simulink model "highpass"  (Simulink 7.7)
settings: Solver=ode45  StartTime=0.0  StopTime=(m-n)*sample  RelTol=1e-3
InitFcn:
  | %% DSPBuilder Start
  | alt_dspbuilder_update_model(bdroot)
  | %% DSPBuilder End
values from neighbouring files (symbols this model uses):
  sample = 10e-9    (= 1e-08)    [readdata.m]
undefined symbols (not defined in the file or in its folder): G, SOS
libraries: allblocks_alteradspbuilder2 x32, simulink x4
settings Model: Creator=Lyq  LastModifiedBy=xj

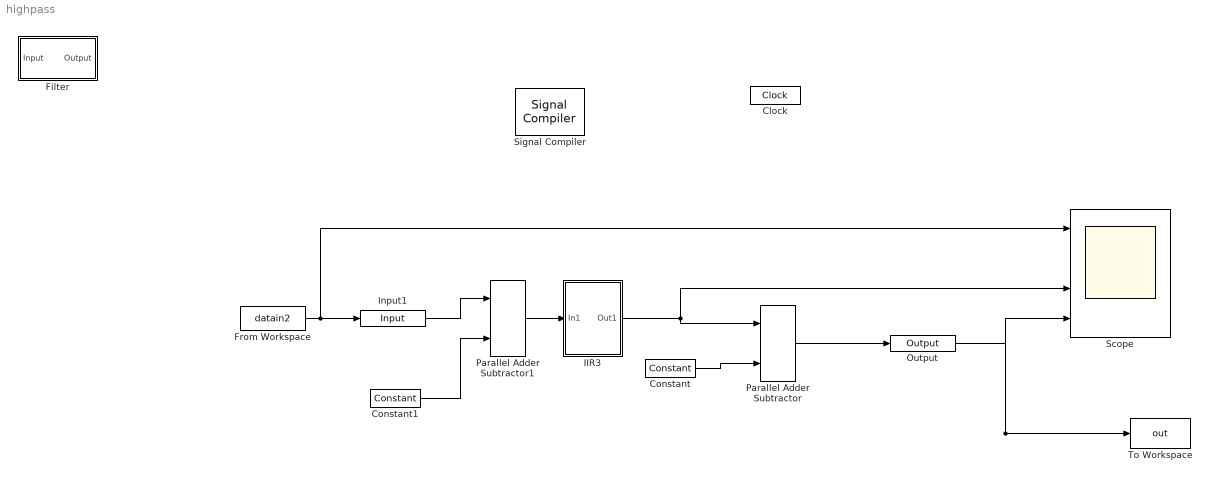
== system highpass ==
  Clock : allblocks_alteradspbuilder2/Clock  ClockPeriod=10  ClockPeriodUnit=ns  SampleTime=10e-9  ResetLatency=0  ResetRegisterCascadeDepth=0  SimulationStartCycle=5  PhaseOffset=0  Reset=aclr  ResetType=Active Low  Export=off
  Constant : allblocks_alteradspbuilder2/Constant  mask_cst=512  BusType=Unsigned Integer  bwl=10  bwr=0  roundMode=Truncate  satMode=Wrap  SpecifyClock=off  allowFloatingPointOverride=on  logOutputs=off  logFile=D:\highpass_Constant.fixedpointlog
  Constant1 : allblocks_alteradspbuilder2/Constant  mask_cst=512  BusType=Unsigned Integer  bwl=10  bwr=0  roundMode=Truncate  satMode=Wrap  SpecifyClock=off  allowFloatingPointOverride=on  logOutputs=off  logFile=D:\highpass_Constant1.fixedpointlog
  Filter : Subsystem  Tag=FilterWizardSubSystem
      settings: ErrorFcn=dspFilterRealizedInBasicElemsAlgLoopErrFcnCallback
  From Workspace : FromWorkspace  VariableName=datain2  SampleTime=sample
  IIR3 : Subsystem
  Input1 : allblocks_alteradspbuilder2/Input  iofile=F:\matlab\DSPbuilder\HighPass(1Mfc-100fs)\tb_highpass\highpass_Input1.salt  BusType=Unsigned Integer  bwl=10  bwr=5  SpecifyClock=off  PORTTYPE=Input  externalType=Inferred  allowFloatingPointOverride=on  logOutputs=off
  Output : allblocks_alteradspbuilder2/Output  iofile=F:\matlab\DSPbuilder\HighPass(1Mfc-100fs)\tb_highpass\highpass_Output.capture  BusType=Unsigned Integer  bwl=10  bwr=0  externalType=Inferred  PORTTYPE=Output  allowFloatingPointOverride=on  logOutputs=off
  Parallel Adder Subtractor : allblocks_alteradspbuilder2/Parallel Adder Subtractor  number_of_inputs=2  direction=+  use_pipeline=on  pipeline_display=1  phase_selection=1  use_ena=off  use_aclr=off  allowFloatingPointOverride=on  logOutputs=off  logFile=F:\matlab\DSPbuilder\bandpass(1-10M)\tb_bandpass\highpass_Parallel+Adder+Subtractor.fixedpointlog
  Parallel Adder Subtractor1 : allblocks_alteradspbuilder2/Parallel Adder Subtractor  number_of_inputs=2  direction=+-  use_pipeline=on  pipeline_display=1  phase_selection=1  use_ena=off  use_aclr=off  allowFloatingPointOverride=on  logOutputs=off  logFile=F:\matlab\DSPbuilder\bandpass(1-10M)\tb_bandpass\highpass_Parallel+Adder+Subtractor1.fixedpointlog
  Scope : Scope  NumInputPorts=4
      settings: TimeRange=3.839999999999997e-006  YMin=-30000~-30000~-40000~-40000  YMax=30000~30000~40000~40000  MaxDataPoints=50000  SampleInput=on
  Signal Compiler : allblocks_alteradspbuilder2/Signal Compiler  DeviceFamily=Cyclone III  DeviceName=AUTO  EnableSignalTap=off  SignalTapDepth=128  UseBoardBlock=off  StpUseDefaultClock=on  StpClock=Clock  ExportDir=F:\matlab\DSPbuilder\bandpass(1-10M)\HDL
  To Workspace : ToWorkspace  VariableName=out  SampleTime=-1  SaveFormat=Structure
  wires:
  From Workspace/1 -> Scope/1, Input1/1
  IIR3/1(Out1) -> Scope/3, Parallel Adder Subtractor/1
  Output/1 -> Scope/4, To Workspace/1
  Constant/1 -> Parallel Adder Subtractor/2
  Parallel Adder Subtractor/1 -> Output/1
  Parallel Adder Subtractor1/1 -> IIR3/1(In1)
  Input1/1 -> Parallel Adder Subtractor1/1
  Constant1/1 -> Parallel Adder Subtractor1/2

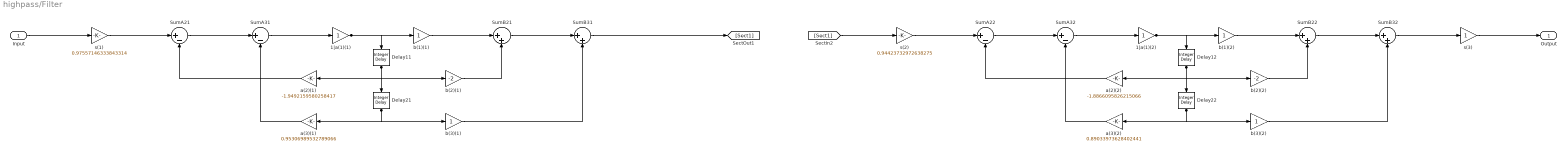
== system highpass/Filter ==
  Input : Inport
  1|a(1)(1) : Gain  ParamDataTypeStr=float('double')  RndMeth=Nearest  SaturateOnIntegerOverflow=on  OutDataTypeStr=Inherit: Same as input
  1|a(1)(2) : Gain  ParamDataTypeStr=float('double')  RndMeth=Nearest  SaturateOnIntegerOverflow=on  OutDataTypeStr=Inherit: Same as input
  Delay{11..12,21..22} (4 alike) : simulink/Discrete/Integer Delay  NumDelays=1  InputProcessing=Inherited  vinit=0  samptime=-1
  SumA{21..22,31..32} (4 alike) : Sum  Inputs=|+-  RndMeth=Nearest  SaturateOnIntegerOverflow=on  OutDataTypeStr=Inherit: Same as first input
  SumB{21..22,31..32} (4 alike) : Sum  Inputs=|++  RndMeth=Nearest  SaturateOnIntegerOverflow=on  OutDataTypeStr=Inherit: Same as first input
  a(2)(1) : Gain  Gain=-1.9492159580258417  ParamDataTypeStr=float('double')  RndMeth=Nearest  SaturateOnIntegerOverflow=on  OutDataTypeStr=Inherit: Same as input
  a(2)(2) : Gain  Gain=-1.8866095826215066  ParamDataTypeStr=float('double')  RndMeth=Nearest  SaturateOnIntegerOverflow=on  OutDataTypeStr=Inherit: Same as input
  a(3)(1) : Gain  Gain=0.95306989532789066  ParamDataTypeStr=float('double')  RndMeth=Nearest  SaturateOnIntegerOverflow=on  OutDataTypeStr=Inherit: Same as input
  a(3)(2) : Gain  Gain=0.89033973628402441  ParamDataTypeStr=float('double')  RndMeth=Nearest  SaturateOnIntegerOverflow=on  OutDataTypeStr=Inherit: Same as input
  b(1)(1) : Gain  ParamDataTypeStr=float('double')  RndMeth=Nearest  SaturateOnIntegerOverflow=on  OutDataTypeStr=Inherit: Same as input
  b(1)(2) : Gain  ParamDataTypeStr=float('double')  RndMeth=Nearest  SaturateOnIntegerOverflow=on  OutDataTypeStr=Inherit: Same as input
  b(2)(1) : Gain  Gain=-2  ParamDataTypeStr=float('double')  RndMeth=Nearest  SaturateOnIntegerOverflow=on  OutDataTypeStr=Inherit: Same as input
  b(2)(2) : Gain  Gain=-2  ParamDataTypeStr=float('double')  RndMeth=Nearest  SaturateOnIntegerOverflow=on  OutDataTypeStr=Inherit: Same as input
  b(3)(1) : Gain  ParamDataTypeStr=float('double')  RndMeth=Nearest  SaturateOnIntegerOverflow=on  OutDataTypeStr=Inherit: Same as input
  b(3)(2) : Gain  ParamDataTypeStr=float('double')  RndMeth=Nearest  SaturateOnIntegerOverflow=on  OutDataTypeStr=Inherit: Same as input
  s(1) : Gain  Gain=0.97557146333843314  ParamDataTypeStr=float('double')  RndMeth=Nearest  SaturateOnIntegerOverflow=on  OutDataTypeStr=Inherit: Same as input
  s(2) : Gain  Gain=0.94423732972638275  ParamDataTypeStr=float('double')  RndMeth=Nearest  SaturateOnIntegerOverflow=on  OutDataTypeStr=Inherit: Same as input
  s(3) : Gain  ParamDataTypeStr=float('double')  RndMeth=Nearest  SaturateOnIntegerOverflow=on  OutDataTypeStr=Inherit: Same as input
  Output : Outport
  wires:
  Input/1 -> s(1)/1
  s(1)/1 -> SumA21/1
  SumA21/1 -> SumA31/1
  SumA31/1 -> 1|a(1)(1)/1
  1|a(1)(1)/1 -> b(1)(1)/1, Delay11/1
  b(1)(1)/1 -> SumB21/1
  SumB21/1 -> SumB31/1
  SumB31/1 -> [Sect1]
  a(2)(1)/1 -> SumA21/2
  Delay11/1 -> a(2)(1)/1, b(2)(1)/1, Delay21/1
  b(2)(1)/1 -> SumB21/2
  a(3)(1)/1 -> SumA31/2
  Delay21/1 -> a(3)(1)/1, b(3)(1)/1
  b(3)(1)/1 -> SumB31/2
  [Sect1] -> s(2)/1
  s(2)/1 -> SumA22/1
  SumA22/1 -> SumA32/1
  SumA32/1 -> 1|a(1)(2)/1
  1|a(1)(2)/1 -> b(1)(2)/1, Delay12/1
  b(1)(2)/1 -> SumB22/1
  SumB22/1 -> SumB32/1
  SumB32/1 -> s(3)/1
  a(2)(2)/1 -> SumA22/2
  Delay12/1 -> a(2)(2)/1, b(2)(2)/1, Delay22/1
  b(2)(2)/1 -> SumB22/2
  a(3)(2)/1 -> SumA32/2
  Delay22/1 -> a(3)(2)/1, b(3)(2)/1
  b(3)(2)/1 -> SumB32/2
  s(3)/1 -> Output/1

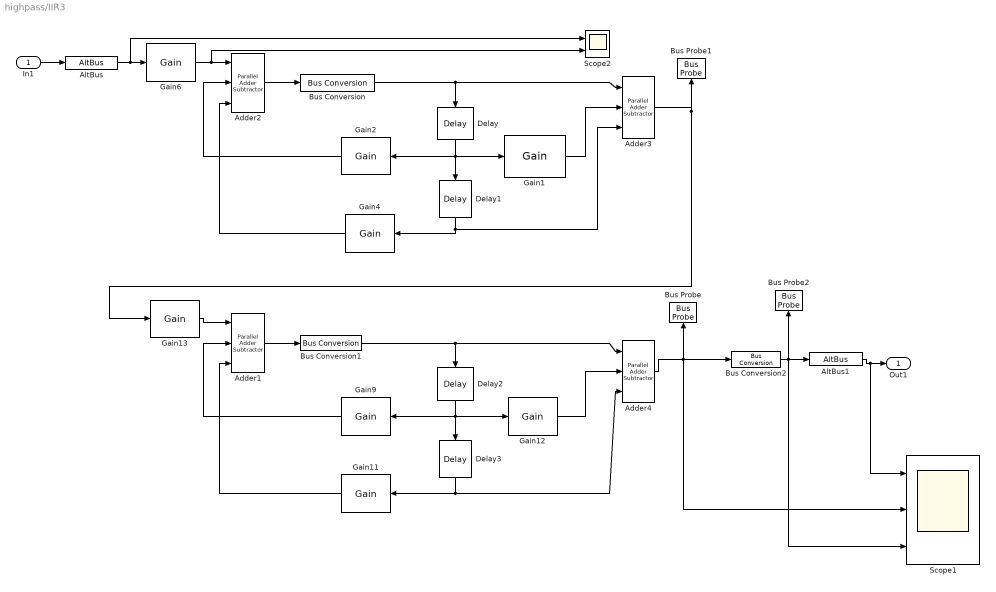
== system highpass/IIR3 ==
  In1 : Inport
  Adder1 : allblocks_alteradspbuilder2/Parallel Adder Subtractor  number_of_inputs=3  direction=+--  use_pipeline=off  pipeline_display=0  phase_selection=1  use_ena=off  use_aclr=off  allowFloatingPointOverride=on  logOutputs=off  logFile=D:\highpass_IIR3_Adder1.fixedpointlog
  Adder2 : allblocks_alteradspbuilder2/Parallel Adder Subtractor  number_of_inputs=3  direction=+--  use_pipeline=off  pipeline_display=0  phase_selection=1  use_ena=off  use_aclr=off  allowFloatingPointOverride=on  logOutputs=off  logFile=D:\highpass_IIR3_Adder2.fixedpointlog
  Adder3 : allblocks_alteradspbuilder2/Parallel Adder Subtractor  number_of_inputs=3  direction=+  use_pipeline=on  pipeline_display=2  phase_selection=1  use_ena=off  use_aclr=off  allowFloatingPointOverride=on  logOutputs=off  logFile=D:\highpass_IIR3_Adder3.fixedpointlog
  Adder4 : allblocks_alteradspbuilder2/Parallel Adder Subtractor  number_of_inputs=3  direction=+  use_pipeline=on  pipeline_display=2  phase_selection=1  use_ena=off  use_aclr=off  allowFloatingPointOverride=on  logOutputs=off  logFile=D:\highpass_IIR3_Adder4.fixedpointlog
  AltBus : allblocks_alteradspbuilder2/AltBus  BusType=Signed Integer  bwl=10  bwr=5  saturate=off  floatingPointInput=on  floatingPointOutput=on  logOutputs=off  logFile=D:\highpass_IIR3_AltBus.fixedpointlog
  AltBus1 : allblocks_alteradspbuilder2/AltBus  BusType=Signed Integer  bwl=10  bwr=5  saturate=on  floatingPointInput=on  floatingPointOutput=on  logOutputs=off  logFile=D:\highpass_IIR3_AltBus1.fixedpointlog
  Bus Conversion : allblocks_alteradspbuilder2/Bus Conversion  BusType=Signed Fractional  ibwl=20  ibwr=5  bwl=20  bwr=5  bitToConnectToOutputLSB=0  round=off  saturate=on  pipeline_display=0
  Bus Conversion1 : allblocks_alteradspbuilder2/Bus Conversion  BusType=Signed Fractional  ibwl=24  ibwr=5  bwl=24  bwr=5  bitToConnectToOutputLSB=0  round=off  saturate=on  pipeline_display=0
  Bus Conversion2 : allblocks_alteradspbuilder2/Bus Conversion  BusType=Signed Integer  ibwl=11  ibwr=1  bwl=10  bwr=1  bitToConnectToOutputLSB=0  round=off  saturate=on  pipeline_display=0
  Bus Probe : allblocks_alteradspbuilder2/Bus Probe  display=Maximum number of integer bits required during simulation  max_value=598.21875  min_value=-618.875  max_bits=11
  Bus Probe1 : allblocks_alteradspbuilder2/Bus Probe  display=Maximum number of integer bits required during simulation  max_value=755.5625  min_value=-665.78125  max_bits=11
  Bus Probe2 : allblocks_alteradspbuilder2/Bus Probe  display=Maximum number of integer bits required during simulation  max_value=511  min_value=-512  max_bits=10
  Delay : allblocks_alteradspbuilder2/Delay  pipeline=1  pipeline_display=1  ClockPhase=1  use_ena=off  use_sclr=off  allowFloatingPointOverride=on  logOutputs=off  logFile=D:\highpass_IIR3_Delay.fixedpointlog  use_init=off  reset_value=1
  Delay1 : allblocks_alteradspbuilder2/Delay  pipeline=1  pipeline_display=1  ClockPhase=1  use_ena=off  use_sclr=off  allowFloatingPointOverride=on  logOutputs=off  logFile=D:\highpass_IIR3_Delay1.fixedpointlog  use_init=off  reset_value=1
  Delay2 : allblocks_alteradspbuilder2/Delay  pipeline=1  pipeline_display=1  ClockPhase=1  use_ena=off  use_sclr=off  allowFloatingPointOverride=on  logOutputs=off  logFile=D:\highpass_IIR3_Delay2.fixedpointlog  use_init=off  reset_value=1
  Delay3 : allblocks_alteradspbuilder2/Delay  pipeline=1  pipeline_display=1  ClockPhase=1  use_ena=off  use_sclr=off  allowFloatingPointOverride=on  logOutputs=off  logFile=D:\highpass_IIR3_Delay3.fixedpointlog  use_init=off  reset_value=1
  Gain1 : allblocks_alteradspbuilder2/Gain  vgain=SOS(1,2)  BusType=Signed Fractional  bwl=2  bwr=16  pipeline=0  pipeline_display=0  allowFloatingPointOverride=on  logOutputs=off  logFile=D:\highpass_IIR3_Gain1.fixedpointlog  use_ena=off  use_aclr=off  lpm=off  MaskValue=1
  Gain11 : allblocks_alteradspbuilder2/Gain  vgain=SOS(2,6)  BusType=Signed Fractional  bwl=2  bwr=10  pipeline=0  pipeline_display=0  allowFloatingPointOverride=on  logOutputs=off  logFile=D:\highpass_IIR3_Gain11.fixedpointlog  use_ena=off  use_aclr=off  lpm=off  MaskValue=1
  Gain12 : allblocks_alteradspbuilder2/Gain  vgain=SOS(2,2)  BusType=Signed Integer  bwl=2  bwr=10  pipeline=0  pipeline_display=0  allowFloatingPointOverride=on  logOutputs=off  logFile=D:\highpass_IIR3_Gain12.fixedpointlog  use_ena=off  use_aclr=off  lpm=off  MaskValue=1
  Gain13 : allblocks_alteradspbuilder2/Gain  vgain=G(2)  BusType=Signed Fractional  bwl=2  bwr=10  pipeline=0  pipeline_display=0  allowFloatingPointOverride=on  logOutputs=off  logFile=D:\highpass_IIR3_Gain13.fixedpointlog  use_ena=off  use_aclr=off  lpm=off  MaskValue=1
  Gain2 : allblocks_alteradspbuilder2/Gain  vgain=SOS(1,5)  BusType=Signed Fractional  bwl=2  bwr=16  pipeline=0  pipeline_display=0  allowFloatingPointOverride=on  logOutputs=off  logFile=D:\highpass_IIR3_Gain2.fixedpointlog  use_ena=off  use_aclr=off  lpm=off  MaskValue=1
  Gain4 : allblocks_alteradspbuilder2/Gain  vgain=SOS(1,6)  BusType=Signed Fractional  bwl=2  bwr=16  pipeline=0  pipeline_display=0  allowFloatingPointOverride=on  logOutputs=off  logFile=D:\highpass_IIR3_Gain4.fixedpointlog  use_ena=off  use_aclr=off  lpm=off  MaskValue=1
  Gain6 : allblocks_alteradspbuilder2/Gain  vgain=G(1)  BusType=Signed Fractional  bwl=2  bwr=16  pipeline=0  pipeline_display=0  allowFloatingPointOverride=on  logOutputs=off  logFile=D:\highpass_IIR3_Gain6.fixedpointlog  use_ena=off  use_aclr=off  lpm=off  MaskValue=1
  Gain9 : allblocks_alteradspbuilder2/Gain  vgain=SOS(2,5)  BusType=Signed Fractional  bwl=2  bwr=10  pipeline=0  pipeline_display=0  allowFloatingPointOverride=on  logOutputs=off  logFile=D:\highpass_IIR3_Gain9.fixedpointlog  use_ena=off  use_aclr=off  lpm=off  MaskValue=1
  Scope1 : Scope  NumInputPorts=3
      settings: TimeRange=7.680000000000001e-006  YMin=-40000~-100000~-100000  YMax=30000~150000~80000  SaveName=ScopeData2
  Scope2 : Scope  NumInputPorts=2
      settings: TimeRange=1  YMin=-5~0  YMax=5~1  SaveName=ScopeData3
  Out1 : Outport
  wires:
  Delay/1 -> Delay1/1, Gain2/1, Gain1/1
  Delay1/1 -> Gain4/1, Adder3/3
  Gain6/1 -> Adder2/1, Scope2/2
  Gain2/1 -> Adder2/2
  Gain4/1 -> Adder2/3
  Adder2/1 -> Bus Conversion/1
  Delay2/1 -> Delay3/1, Gain9/1, Gain12/1
  Delay3/1 -> Gain11/1, Adder4/3
  Gain13/1 -> Adder1/1
  Gain9/1 -> Adder1/2
  Gain11/1 -> Adder1/3
  Adder1/1 -> Bus Conversion1/1
  In1/1 -> AltBus/1
  AltBus1/1 -> Out1/1, Scope1/1
  AltBus/1 -> Gain6/1, Scope2/1
  Adder4/1 -> Scope1/2, Bus Probe/1, Bus Conversion2/1
  Gain1/1 -> Adder3/2
  Gain12/1 -> Adder4/2
  Bus Conversion1/1 -> Delay2/1, Adder4/1
  Bus Conversion/1 -> Delay/1, Adder3/1
  Adder3/1 -> Bus Probe1/1, Gain13/1
  Bus Conversion2/1 -> AltBus1/1, Bus Probe2/1, Scope1/3
